simulink model "Lab3"  (Simulink 8.6)
settings: Solver=VariableStepAuto  StartTime=0.0  StopTime=10.0  RelTol=1e-3
values from neighbouring files (symbols this model uses):
  k1 = double(gains.k1)    [MTRE4010_Assignment.m]
  k2 = double(gains.k2)    [MTRE4010_Assignment.m]
undefined symbols (not defined in the file or in its folder): k3, m1, m2
libraries: simulink_extras x1
settings Model: Creator=Jacques-Ezechiel  LastModifiedBy=Jacques-Ezechiel
settings DataIOCC: SaveFormat=Dataset  SignalLoggingSaveFormat=Dataset
settings OptimizationCC: ExpressionDepthLimit=128
settings DebuggingCC: UnderspecifiedInitializationDetection=Simplified  MergeDetectMultiDrivingBlocksExec=error  SolverPrmCheckMsg=none  FcnCallInpInsideContextMsg=EnableAllAsError  StateNameClashWarn=none
settings HardwareCC: ProdBitPerPointer=64  ProdLargestAtomicFloat=Float  ProdIntDivRoundTo=Zero  ProdEndianess=LittleEndian  ProdWordSize=64  ProdHWDeviceType=Intel->x86-64 (Windows64)
settings GRTTargetCC: GeneratePreprocessorConditionals=Use local settings  CombineOutputUpdateFcns=on  GRTInterface=off
settings ConfigComp: CovModelRefEnable=off

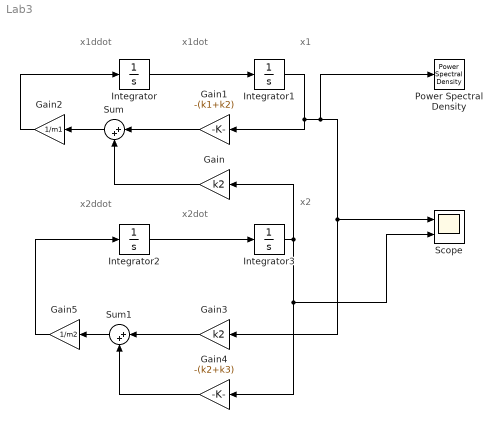
== system Lab3 ==
  note: x1
  note: x1dot
  note: x1ddot
  note: x2ddot
  note: x2dot
  note: x2
  Gain : Gain  Gain=k2
  Gain1 : Gain  Gain=-(k1+k2)
  Gain2 : Gain  Gain=1/m1
  Gain3 : Gain  Gain=k2
  Gain4 : Gain  Gain=-(k2+k3)
  Gain5 : Gain  Gain=1/m2
  Integrator : Integrator
  Integrator1 : Integrator  InitialCondition=.01  LimitOutput=on  UpperSaturationLimit=.03  LowerSaturationLimit=-.03
  Integrator2 : Integrator
  Integrator3 : Integrator  InitialCondition=0.02  LimitOutput=on  UpperSaturationLimit=.03  LowerSaturationLimit=-.03
  Power Spectral Density : simulink_extras/Additional Sinks/Power Spectral Density  npts=128  fftpts=512  HowOften=64  sampleT=0.1
  Scope : Scope  NumInputPorts=2
  Sum : Sum  Inputs=|++
  Sum1 : Sum  Inputs=|++
  wires:
  Integrator/1 -> Integrator1/1
  Integrator2/1 -> Integrator3/1
  Integrator1/1 -> Power Spectral Density/1, Gain3/1, Scope/1, Gain1/1
  Gain/1 -> Sum/2
  Gain1/1 -> Sum/1
  Sum/1 -> Gain2/1
  Gain2/1 -> Integrator/1
  Gain3/1 -> Sum1/1
  Gain4/1 -> Sum1/2
  Integrator3/1 -> Gain4/1, Scope/2, Gain/1
  Sum1/1 -> Gain5/1
  Gain5/1 -> Integrator2/1
